simulink model "Lab_8_Act2"  (R2014a)
settings: Solver=ode23t  StartTime=0.0  StopTime=20  RelTol=1e-3
settings Model: Creator=cloughj  LastModifiedBy=cloughj
settings SolverCC: ZeroCrossAlgorithm=Adaptive

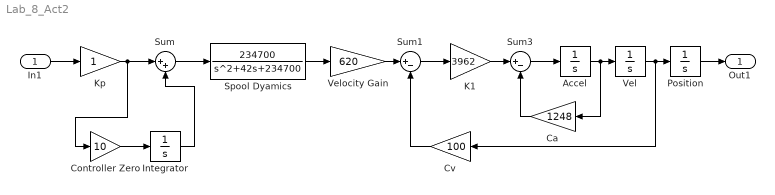
== system Lab_8_Act2 ==
  In1 : Inport
  Accel : Integrator
  Ca : Gain  Gain=1248
  Controller Zero : Gain  Gain=10
  Cv : Gain  Gain=100
  Integrator : Integrator
  K1 : Gain  Gain=3962
  Kp : Gain
  Position : Integrator
  Spool Dyamics : TransferFcn  Numerator=[234700]  Denominator=[1 42 234700]
  Sum : Sum  Inputs=|++
  Sum1 : Sum  Inputs=|+-
  Sum3 : Sum  Inputs=|+-
  Vel : Integrator
  Velocity Gain : Gain  Gain=620
  Out1 : Outport
  wires:
  Velocity Gain/1 -> Sum1/1
  Cv/1 -> Sum1/2
  Kp/1 -> Controller Zero/1, Sum/1
  Sum/1 -> Spool Dyamics/1
  Controller Zero/1 -> Integrator/1
  Integrator/1 -> Sum/2
  Spool Dyamics/1 -> Velocity Gain/1
  Sum1/1 -> K1/1
  K1/1 -> Sum3/1
  Sum3/1 -> Accel/1
  Accel/1 -> Ca/1, Vel/1
  Vel/1 -> Cv/1, Position/1
  Ca/1 -> Sum3/2
  In1/1 -> Kp/1
  Position/1 -> Out1/1
